simulink model "a"  (R2023a)
settings: Solver=ode4  StartTime=0.0  StopTime=400  FixedStep=0.1  RelTol=1e-3
InitFcn:
  | init;
undefined symbols (not defined in the file or in its folder): a_u_lim, gamma_0, L_1, N, V_u, x_0, y_0
settings Model: Creator=Ali  LastModifiedBy=Ali

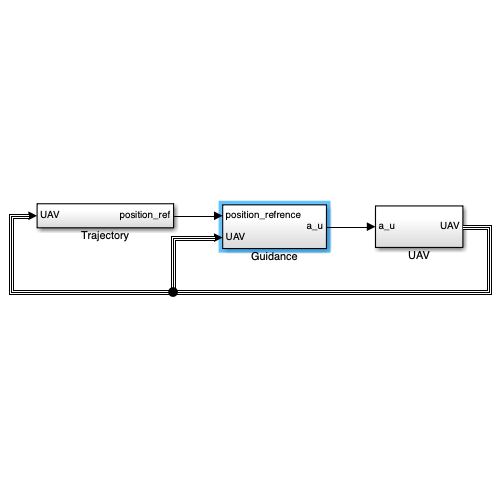
[thumbnail: Simulink's stored preview of the top-level diagram]
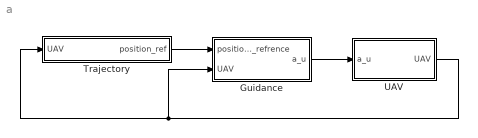
== system a ==
  Guidance : Subsystem
  Trajectory : Subsystem
  UAV : Subsystem
  wires:
  UAV/1(UAV) -> Trajectory/1(UAV), Guidance/2(UAV)
  Guidance/1(a_u) -> UAV/1(a_u)
  Trajectory/1(position_ref) -> Guidance/1(position_refrence)

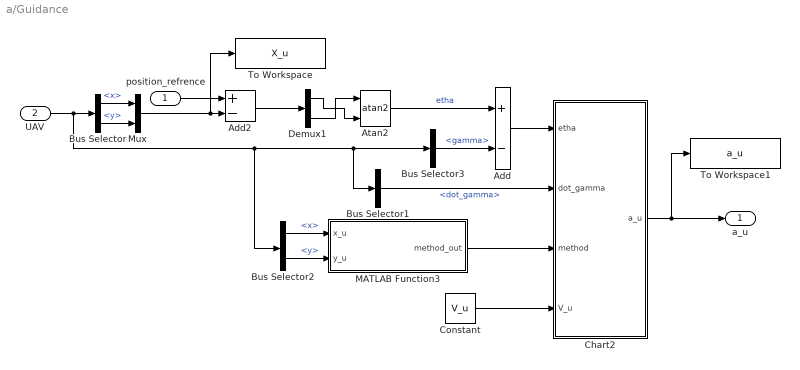
== system a/Guidance ==
  position_refrence : Inport
  UAV : Inport  Port=2
  Add : Sum  Inputs=+-
  Add2 : Sum  Inputs=+-
  Atan2 : Trigonometry  Operator=atan2
  Bus Selector : BusSelector  OutputSignals=x,y
  Bus Selector1 : BusSelector  OutputSignals=dot_gamma
  Bus Selector2 : BusSelector  OutputSignals=x,y
  Bus Selector3 : BusSelector  OutputSignals=gamma
  Chart2 : Stateflow chart  TreatAsAtomicUnit=on
      settings: PortSchema="{\"entries\":[{\"content\":{\"sides\":[{\"content\":{\"connectorIds\":[\"In2\",\"In1\",\"In3\",\"In4\"]},\"type\":\"ConnectorPlacement.EquallySpacedRectSide\",\"uuid\":\"830c4b3f-6595-47a2-a683-b13964dc589e\"},{\"content\":{\"connectorIds\":[\"Out1\"],\"side\":\"RIGHT\"},\"type\":\"ConnectorPlacement.EquallySpacedRectSide\",\"uuid\":\"fc41335a-8bf8-4ed1-8cb1-621fe482d25a\"},{\"content\":{\"side\":\"TOP\"},\"type\":\"ConnectorPlacement.EquallySpacedRectSide\",\"uuid\":\"79c83440-3b91-4923-976e-f1d6a1f3b5ff\"}]},\"type\":\"ConnectorPlacement.EquallySpacedConnector\",\"uuid\":\"f396a7f8-7c0a-40ca-9407-1e850a718b75\"}],\"packageUris\":[\"http://schema.mathworks.com/mf0/Connector/R2020b\"],\"version\":\"1.0\"}"
  Constant : Constant  Value=V_u
  Demux1 : Demux  Outputs=2
  MATLAB Function3 : MATLAB Function  TreatAsAtomicUnit=on
  Mux : Mux  Inputs=2
  To Workspace : ToWorkspace  VariableName=X_u  SaveFormat=Structure With Time  SampleTime=-1
  To Workspace1 : ToWorkspace  VariableName=a_u  SaveFormat=Structure With Time  SampleTime=-1
  a_u : Outport
  wires:
  UAV/1 -> Bus Selector2/1, Bus Selector3/1, Bus Selector1/1, Bus Selector/1
  Bus Selector/2 -> Mux/2  "<y>"
  position_refrence/1 -> Add2/1
  Add2/1 -> Demux1/1
  Mux/1 -> To Workspace/1, Add2/2
  Bus Selector/1 -> Mux/1  "<x>"
  Bus Selector1/1 -> Chart2/1(dot_gamma)  "<dot_gamma>"
  Constant/1 -> Chart2/4(V_u)
  Chart2/1(a_u) -> To Workspace1/1, a_u/1
  MATLAB Function3/1(method_out) -> Chart2/3(method)
  Bus Selector2/1 -> MATLAB Function3/1(x_u)  "<x>"
  Bus Selector2/2 -> MATLAB Function3/2(y_u)  "<y>"
  Atan2/1 -> Add/1  "etha"
  Bus Selector3/1 -> Add/2  "<gamma>"
  Demux1/2 -> Atan2/1
  Demux1/1 -> Atan2/2
  Add/1 -> Chart2/2(etha)

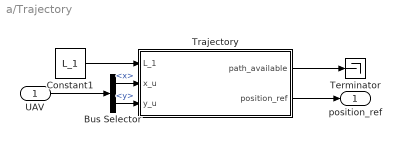
== system a/Trajectory ==
  UAV : Inport
  Bus Selector : BusSelector  OutputSignals=x,y
  Constant1 : Constant  Value=L_1
  Terminator : Terminator
  Trajectory : MATLAB Function  TreatAsAtomicUnit=on
  position_ref : Outport
  wires:
  Trajectory/2(position_ref) -> position_ref/1
  Bus Selector/1 -> Trajectory/2(x_u)  "<x>"
  Trajectory/1(path_available) -> Terminator/1
  UAV/1 -> Bus Selector/1
  Bus Selector/2 -> Trajectory/3(y_u)  "<y>"
  Constant1/1 -> Trajectory/1(L_1)

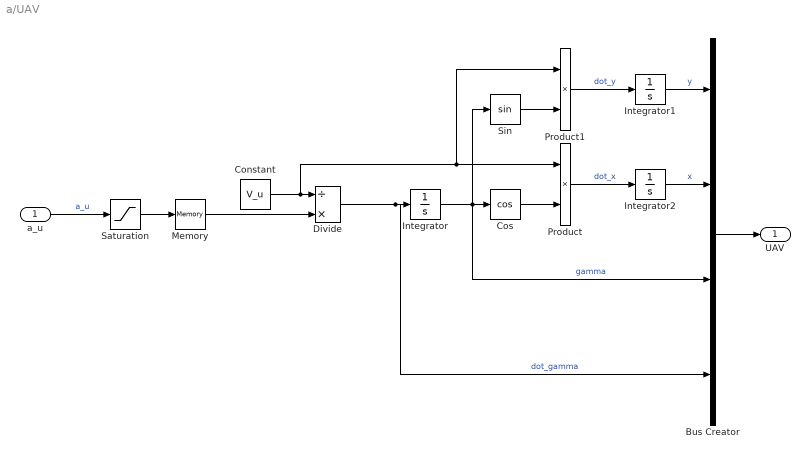
== system a/UAV ==
  a_u : Inport
  Bus Creator : BusCreator  Inputs=4
  Constant : Constant  Value=V_u
  Cos : Trigonometry  Operator=cos
  Divide : Product  Inputs=/*
  Integrator : Integrator  InitialCondition=gamma_0
  Integrator1 : Integrator  InitialCondition=y_0
  Integrator2 : Integrator  InitialCondition=x_0
  Memory : Memory
  Product : Product
  Product1 : Product
  Saturation : Saturate  UpperLimit=a_u_lim  LowerLimit=-a_u_lim
  Sin : Trigonometry
  UAV : Outport
  wires:
  Sin/1 -> Product1/2
  Integrator/1 -> Bus Creator/3, Cos/1, Sin/1  "gamma"
  Integrator2/1 -> Bus Creator/2  "x"
  Product1/1 -> Integrator1/1  "dot_y"
  Product/1 -> Integrator2/1  "dot_x"
  Integrator1/1 -> Bus Creator/1  "y"
  Divide/1 -> Bus Creator/4, Integrator/1  "dot_gamma"
  a_u/1 -> Saturation/1  "a_u"
  Cos/1 -> Product/2
  Constant/1 -> Product/1, Product1/1, Divide/1
  Bus Creator/1 -> UAV/1
  Memory/1 -> Divide/2
  Saturation/1 -> Memory/1

== matlab function a/Trajectory/Trajectory ==
  data: path_available output; L_1 input; position_ref output; x_u input; y_u input
function [path_available, position_ref] = trajectory(L_1, x_u, y_u)



x = 0:1:50000;
x = 50000 - x;
y = 0.5*x;
for i=1:1:length(x)
    if L_1 > sqrt((x(i)-x_u)^2 + (y(i)-y_u)^2)
        path_available = 1;
        break
    else 
        path_available = 0;
    end 
end

position_ref = [x(i), y(i)];

== matlab function a/Guidance/MATLAB Function3 ==
  settings: updateMethod=DISCRETE
  data: x_u input; method_out output; y_u input; L_1 parameter
function method_out = ref_distance(x_u,y_u, L_1)

persistent method
if isempty(method)
    method = 1;
end
ref_dis = (x_u^2 + y_u^2)^0.5;
if ref_dis<0.8*L_1
    method = 2;
end
method_out = method;

== stateflow chart a/Guidance/Chart2 ==
  state PPN
    a_u = N*V_u*dot_gamma;
  state Nonlinear_Guidance_Algorithm
    a_u =  V_u^2*sin(etha)/L_1;
  (default) -> PPN
  PPN -> Nonlinear_Guidance_Algorithm : [method == 2]
  data: dot_gamma input; etha input; method input; a_u output; V_u input; N parameter; L_1 parameter
